simulink model "PID_left_wheels"  (R2017b)
settings: Solver=ode4  StartTime=0.0  StopTime=50  FixedStep=0.01  RelTol=1e-6  EnableMultiTasking=on
settings Model: Creator=Rafael  LastModifiedBy=root
settings DataIOCC: LimitDataPoints=on  SaveFormat=Array
settings OptimizationCC: LifeSpan=inf
settings DebuggingCC: SFUnexpectedBacktrackingDiag=warning  SFNoUnconditionalDefaultTransitionDiag=warning  SFExecutionAtInitializationDiag=none
settings HardwareCC: ProdBitPerPointer=32  ProdBitPerSizeT=32  ProdBitPerPtrDiffT=32  ProdLargestAtomicFloat=None  ProdIntDivRoundTo=Undefined  ProdEndianess=Unspecified  ProdWordSize=32  ProdHWDeviceType=32-bit Generic
settings ModelReferenceCC: PropagateSignalLabelsOutOfModel=off
settings CodeAppCC: StateflowObjectComments=on
settings GRTTargetCC: TargetLangStandard=C89/C90 (ANSI)  GeneratePreprocessorConditionals=Disable all
settings ConfigComp: CovMetricSettings=dw  CovHtmlReporting=on  CovSaveCumulativeToWorkspaceVar=on  CovSaveSingleToWorkspaceVar=on  CovExternalEMLEnable=off

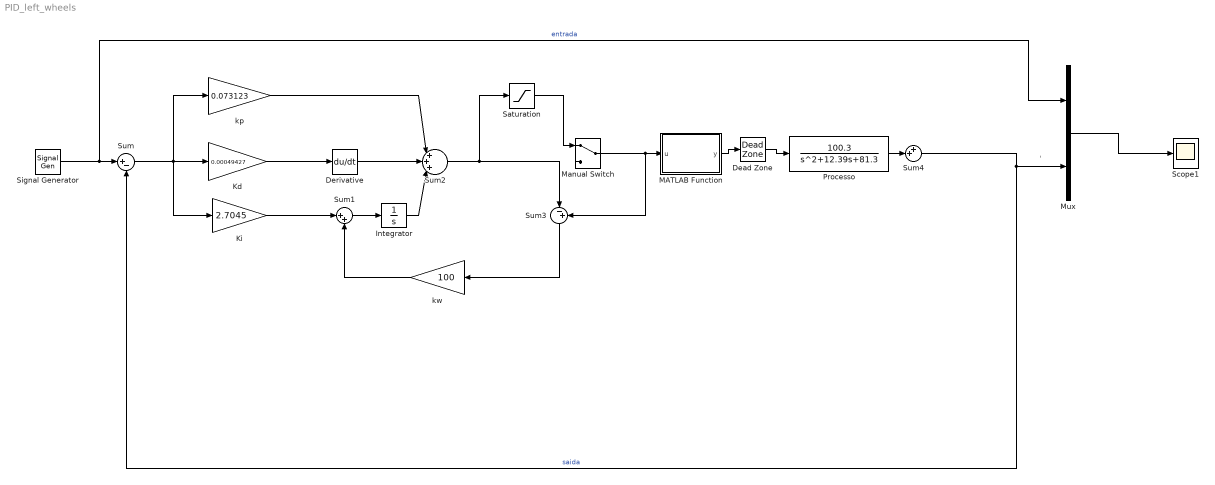
== system PID_left_wheels ==
  note: '
  Dead Zone : DeadZone  LowerValue=-1  UpperValue=1  SaturateOnIntegerOverflow=on
  Derivative : Derivative
  Integrator : Integrator
  Kd : Gain  Gain=0.00049427
  Ki : Gain  Gain=2.7045
  MATLAB Function : MATLAB Function  TreatAsAtomicUnit=on
  Manual Switch : ManualSwitch
  Mux : Mux  Inputs=2
  Processo : TransferFcn  Numerator=[100.3]  Denominator=[1 12.39 81.3]
  Saturation : Saturate  UpperLimit=6  LowerLimit=-6
  Scope1 : Scope
  Signal Generator : SignalGenerator  WaveForm=square  Amplitude=7  Frequency=0.08
  Sum : Sum  Inputs=|+-
  Sum1 : Sum  Inputs=|++
  Sum2 : Sum  Inputs=|+++|
  Sum3 : Sum  Inputs=|-+
  Sum4 : Sum  Inputs=++|
  kp : Gain  Gain=0.073123
  "kw " : Gain  Gain=100
  wires:
  Dead Zone/1 -> Processo/1
  Sum/1 -> kp/1, Kd/1, Ki/1
  kp/1 -> Sum2/1
  Derivative/1 -> Sum2/2
  Sum1/1 -> Integrator/1
  Integrator/1 -> Sum2/3
  Manual Switch/1 -> MATLAB Function/1(u), Sum3/2
  Saturation/1 -> Manual Switch/1
  Sum4/1 -> Sum/2, Mux/2  "saida"
  Processo/1 -> Sum4/2
  Signal Generator/1 -> Mux/1, Sum/1  "entrada"
  Kd/1 -> Derivative/1
  MATLAB Function/1(y) -> Dead Zone/1
  Ki/1 -> Sum1/1
  "kw "/1 -> Sum1/2
  Mux/1 -> Scope1/1
  Sum3/1 -> "kw "/1
  Sum2/1 -> Sum3/1, Saturation/1

== matlab function PID_left_wheels/MATLAB Function ==
  data: u input; y output
function y = inverte(u)
if (u > 0)
    u = u + 1;
end 
if (u <= 0)
    u = u - 1;
end 
y = u;
